simulink model "MLPQ3"  (R2022b)
settings: Solver=VariableStepAuto  StartTime=0.0  StopTime=500  RelTol=1e-3
settings Model: Creator=Mojtaba  LastModifiedBy=AVAJANG
settings ModelReferenceCC: EnableRefExpFcnMdlSchedulingChecks=on

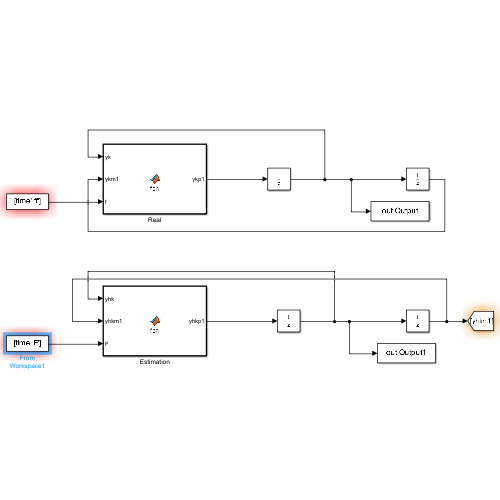
[thumbnail: Simulink's stored preview of the top-level diagram]
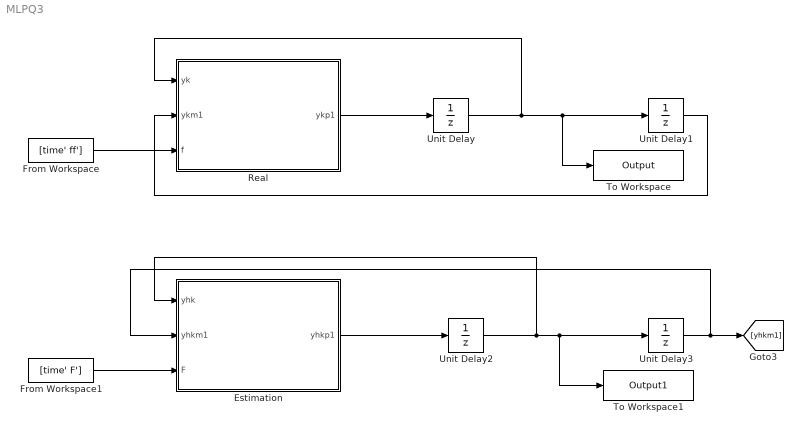
== system MLPQ3 ==
  Estimation : MATLAB Function  TreatAsAtomicUnit=on
  From Workspace : FromWorkspace  VariableName=[time' ff']
  From Workspace1 : FromWorkspace  VariableName=[time' F']
  Real : MATLAB Function  TreatAsAtomicUnit=on
  To Workspace : ToWorkspace  VariableName=Output  SaveFormat=Timeseries  SampleTime=-1
  To Workspace1 : ToWorkspace  VariableName=Output1  SaveFormat=Timeseries  SampleTime=-1
  Unit Delay{,1..3} (4 alike) : UnitDelay  HasFrameUpgradeWarning=on
  wires:
  Unit Delay/1 -> Real/1(yk), To Workspace/1, Unit Delay1/1
  Unit Delay1/1 -> Real/2(ykm1)
  Unit Delay2/1 -> Unit Delay3/1, To Workspace1/1, Estimation/1(yhk)
  Unit Delay3/1 -> Estimation/2(yhkm1), [yhkm1]
  From Workspace/1 -> Real/3(f)
  From Workspace1/1 -> Estimation/3(F)
  Real/1(ykp1) -> Unit Delay/1
  Estimation/1(yhkp1) -> Unit Delay2/1

== matlab function MLPQ3/Real ==
  data: yk input; ykp1 output; ykm1 input; f input
function ykp1 = fcn(yk,ykm1,f)

ykp1=0.3*yk + 0.6*ykm1 + f;

end

== matlab function MLPQ3/Estimation ==
  data: yhk input; yhkp1 output; yhkm1 input; F input
function yhkp1 = fcn(yhk,yhkm1,F)

yhkp1=0.3*yhk + 0.6*yhkm1 + F;

end
